simulink model "Saturation"  (R2025b)
settings: Solver=FixedStepDiscrete  StartTime=0.0  StopTime=10.0  FixedStep=0.01  RelTol=1e-3
libraries: simulink x2
settings Model: Creator=soura  LastModifiedBy=soura

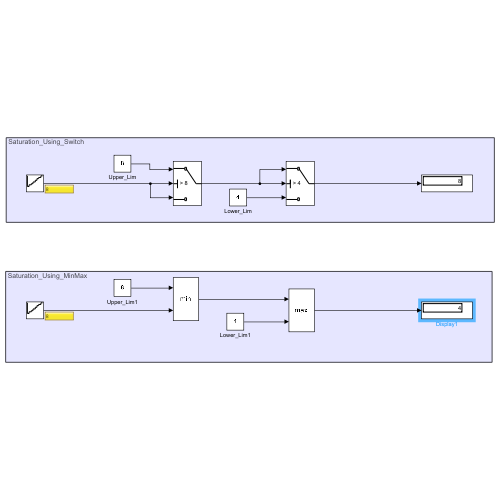
[thumbnail: Simulink's stored preview of the top-level diagram]
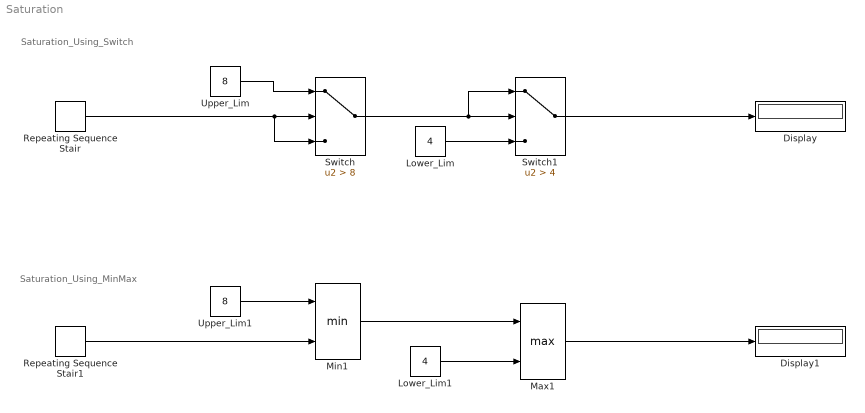
== system Saturation ==
  note: Saturation_Using_MinMax
  note: Saturation_Using_Switch
  Display : Display
  Display1 : Display
  Lower_Lim : Constant  Value=4
  Lower_Lim1 : Constant  Value=4
  Max1 : MinMax  Function=max  Inputs=2
  Min1 : MinMax  Inputs=2
  Repeating Sequence Stair : simulink/Sources/Repeating Sequence Stair  OutValues=[2 3 4 5 6 7 8 9].'  tsamp=-1  OutMin=[]  OutMax=[]  OutDataTypeStr=double  OutputDataTypeScalingMode=double  OutDataType=fixdt(0,8)  ConRadixGroup=Best Precision: Vector-wise  OutScaling=2^-12
  Repeating Sequence Stair1 : simulink/Sources/Repeating Sequence Stair  OutValues=[2 3 4 5 6 7 8 9].'  tsamp=-1  OutMin=[]  OutMax=[]  OutDataTypeStr=double  OutputDataTypeScalingMode=double  OutDataType=fixdt(0,8)  ConRadixGroup=Best Precision: Vector-wise  OutScaling=2^-12
  Switch : Switch  Criteria=u2 > Threshold  Threshold=8  SaturateOnIntegerOverflow=off  InputSameDT=off
  Switch1 : Switch  Criteria=u2 > Threshold  Threshold=4  SaturateOnIntegerOverflow=off  InputSameDT=off
  Upper_Lim : Constant  Value=8
  Upper_Lim1 : Constant  Value=8
  wires:
  Switch/1 -> Switch1/1, Switch1/2
  Upper_Lim/1 -> Switch/1
  Lower_Lim/1 -> Switch1/3
  Repeating Sequence Stair/1 -> Switch/3, Switch/2
  Switch1/1 -> Display/1
  Repeating Sequence Stair1/1 -> Min1/2
  Upper_Lim1/1 -> Min1/1
  Min1/1 -> Max1/1
  Lower_Lim1/1 -> Max1/2
  Max1/1 -> Display1/1
